simulink model "friction_function"  (R2020b)
settings: Solver=VariableStepAuto  StartTime=0.0  StopTime=10.0  RelTol=1e-3
settings Model: Creator=Bens PC  LastModifiedBy=jonas

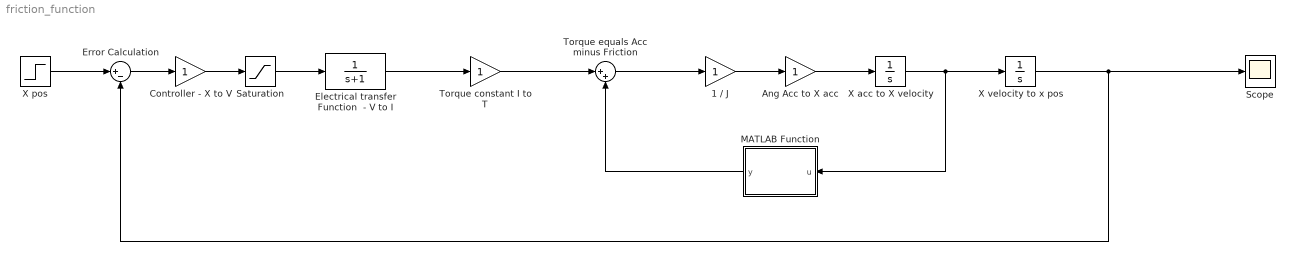
== system friction_function ==
  1 / J : Gain
  Ang Acc to X acc : Gain
  Controller - X to V : Gain
  Electrical transfer Function  - V to I : TransferFcn  Denominator=[1 1]
  Error Calculation : Sum  Inputs=|+-
  MATLAB Function : MATLAB Function  TreatAsAtomicUnit=on
  Saturation : Saturate
  Scope : Scope
  "Torque constant I to T " : Gain
  Torque equals Acc minus Friction : Sum  Inputs=|++
  X acc to X velocity : Integrator
  X pos : Step  SampleTime=0
  X velocity to x pos : Integrator
  wires:
  Error Calculation/1 -> Controller - X to V/1
  Electrical transfer Function  - V to I/1 -> "Torque constant I to T "/1
  "Torque constant I to T "/1 -> Torque equals Acc minus Friction/1
  Torque equals Acc minus Friction/1 -> 1 / J/1
  1 / J/1 -> Ang Acc to X acc/1
  Ang Acc to X acc/1 -> X acc to X velocity/1
  X acc to X velocity/1 -> MATLAB Function/1(u), X velocity to x pos/1
  X pos/1 -> Error Calculation/1
  Controller - X to V/1 -> Saturation/1
  Saturation/1 -> Electrical transfer Function  - V to I/1
  X velocity to x pos/1 -> Scope/1, Error Calculation/2
  MATLAB Function/1(y) -> Torque equals Acc minus Friction/2

== matlab function friction_function/MATLAB Function ==
  data: u input; y output
function y = fcn(u)

% For this function, y is friction and u is trasnlational velocity
%The following constants are dependent on the parameters of the system
%They are take from Design of Control Systems Dec 20, 2016
gamma = 749;%  [-]
F_s = 17.5; % [N]
F_v = 13.0; %[N * s * m^-1]
delta = 0.652; % [-]

y = tanh(u * gamma) * F_s + F_v * (abs(u) ^delta);
